simulink model "MIPI"  (R2025a)
settings: Solver=ode1  StartTime=0.0  StopTime=Ttotal  FixedStep=Tsample  MaxStep=1e-3  RelTol=1e-3
values from neighbouring files (symbols this model uses):
  A_0 = 1.5762    [Para_PV.m]
  alpha_T = 0.048/100    (= 0.00048)    [Para_PV.m]
  beta_T = -0.32/100    (= -0.0032)    [Para_PV.m]
  Ee = 1    [Para_PV.m]
  gamma = -0.0528    [Para_PV.m]
  Iscs = Iscs    (= 8.7)    [Para_PV.m]
  Np = 1    [Para_PV.m]
  Ns = 60    [Para_PV.m]
  qk0 = 11594    [Para_PV.m]
  Tc = 25    [Para_PV.m]
  Ttotal = 5e-1    (= 0.5)    [Batch_Run_MIPI.m]
  Vocs = Vocs/Ns    (= 0.623333333333)    [Para_PV.m]
settings Model: Creator=mwxiao  LastModifiedBy=yvenk
settings SolverCC: AlgebraicLoopSolver=TrustRegion
settings DataIOCC: LimitDataPoints=on  SaveFormat=Array  SignalLoggingSaveFormat=ModelDataLogs  ReturnWorkspaceOutputs=off  SignalLoggingName=sigsOut
settings OptimizationCC: ExpressionDepthLimit=2147483647.0  LifeSpan=inf
settings DebuggingCC: SaveWithParameterizedLinksMsg=none  UnderspecifiedInitializationDetection=Classic  MergeDetectMultiDrivingBlocksExec=none  SignalResolutionControl=TryResolveAllWithWarning  MultiTaskDSMMsg=warning  MultiTaskCondExecSysMsg=none  FcnCallInpInsideContextMsg=warning  UnconnectedInputMsg=warning  UnconnectedOutputMsg=warning  UnconnectedLineMsg=warning  StateNameClashWarn=warning  SFUnexpectedBacktrackingDiag=warning  SFNoUnconditionalDefaultTransitionDiag=warning  SFExecutionAtInitializationDiag=none  ArithmeticOperatorsInVariantConditions=warning
settings HardwareCC: ProdBitPerPointer=32.0  ProdBitPerSizeT=32.0  ProdBitPerPtrDiffT=32.0  ProdLargestAtomicFloat=None  ProdIntDivRoundTo=Undefined  ProdEndianess=Unspecified  ProdWordSize=32.0  ProdHWDeviceType=32-bit Generic  TargetBitPerPointer=64.0  TargetBitPerSizeT=64.0  TargetBitPerPtrDiffT=64.0  TargetLongLongMode=on  TargetIntDivRoundTo=Zero  TargetEndianess=LittleEndian  TargetWordSize=64.0  TargetHWDeviceType=MATLAB Host  ProdEqTarget=off
settings ModelReferenceCC: EnableRefExpFcnMdlSchedulingChecks=on  PropagateSignalLabelsOutOfModel=off
settings SFSimCC: SimUseLocalCustomCode=off  CustomCodeUndefinedFunction=UseInterfaceOnly
settings RTWCC: RTWUseLocalCustomCode=off  GPUComputeCapability=3.5  DLArmComputeVersion=19.05
settings CodeAppCC: StateflowObjectComments=on
settings GRTTargetCC: TargetLangStandard=C89/C90 (ANSI)  CombineOutputUpdateFcns=off  GRTInterface=on
settings ConfigComp: CovMetricSettings=dw  CovSaveCumulativeToWorkspaceVar=on  CovSaveSingleToWorkspaceVar=on  CovExternalEMLEnable=off

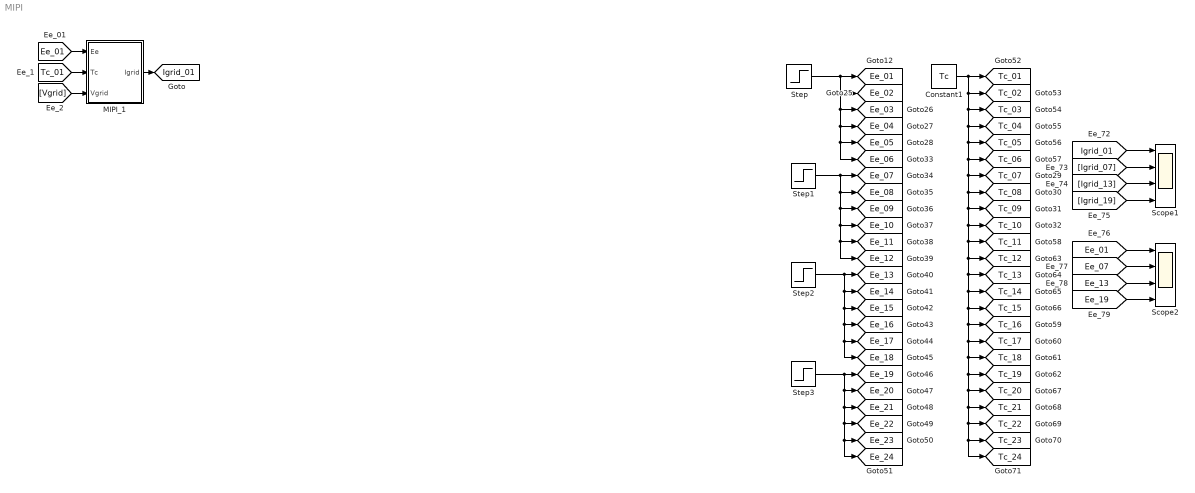
== system MIPI ==
  Constant1 : Constant  Value=Tc
  MIPI_1 : Subsystem
  Scope1 : Scope  NumInputPorts=4
      settings: ActiveDisplayYMinimum=-1.5  ActiveDisplayYMaximum=1.5  DataLoggingVariableName=simout
  Scope2 : Scope  NumInputPorts=4
      settings: ActiveDisplayYMinimum=-1.5  ActiveDisplayYMaximum=1.5  DataLoggingVariableName=simout1
  Step : Step  Time=Ttotal/2+0.005  Before=Ee*0.9  After=Ee*0.7  SampleTime=0
  Step1 : Step  Time=Ttotal/2+0.005  Before=Ee*0.8  After=Ee*0.6  SampleTime=0
  Step2 : Step  Time=Ttotal/2+0.005  Before=Ee*0.7  After=Ee*0.5  SampleTime=0
  Step3 : Step  Time=Ttotal/2+0.005  Before=Ee*0.6  After=Ee*0.8  SampleTime=0
  tag scope: Ee_01=global, Ee_02=global, Ee_03=global, Ee_04=global, Ee_05=global, Ee_06=global, Ee_07=global, Ee_08=global, Ee_09=global, Ee_10=global, Ee_11=global, Ee_12=global, Ee_13=global, Ee_14=global, Ee_15=global, Ee_16=global, Ee_17=global, Ee_18=global, Ee_19=global, Ee_20=global, Ee_21=global, Ee_22=global, Ee_23=global, Ee_24=global, Igrid_01=global, Tc_01=global, Tc_02=global, Tc_03=global, Tc_04=global, Tc_05=global, Tc_06=global, Tc_07=global, Tc_08=global, Tc_09=global, Tc_10=global, Tc_11=global, Tc_12=global, Tc_13=global, Tc_14=global, Tc_15=global, Tc_16=global, Tc_17=global, Tc_18=global, Tc_19=global, Tc_20=global, Tc_21=global, Tc_22=global, Tc_23=global, Tc_24=global
  wires:
  [Ee_13] -> Scope2/3
  [Ee_19] -> Scope2/4
  Step1/1 -> [Ee_11], [Ee_12], [Ee_10], [Ee_09], [Ee_08], [Ee_07]
  [Igrid_13] -> Scope1/3
  [Ee_01] -> Scope2/1
  [Igrid_01] -> Scope1/1
  [Igrid_19] -> Scope1/4
  [Ee_07] -> Scope2/2
  [Igrid_07] -> Scope1/2
  Step/1 -> [Ee_01], [Ee_03], [Ee_04], [Ee_05], [Ee_06], [Ee_02]
  Constant1/1 -> [Tc_08], [Tc_17], [Tc_18], [Tc_21], [Tc_22], [Tc_23], [Tc_24], [Tc_20], [Tc_19], [Tc_16], [Tc_15], [Tc_14], [Tc_13], [Tc_12], [Tc_11], [Tc_10], [Tc_09], [Tc_07], [Tc_06], [Tc_05], [Tc_04], [Tc_03], [Tc_02], [Tc_01]
  Step3/1 -> [Ee_23], [Ee_24], [Ee_22], [Ee_21], [Ee_20], [Ee_19]
  Step2/1 -> [Ee_17], [Ee_18], [Ee_16], [Ee_15], [Ee_14], [Ee_13]
  [Vgrid] -> MIPI_1/3(Vgrid)
  [Tc_01] -> MIPI_1/2(Tc)
  [Ee_01] -> MIPI_1/1(Ee)
  MIPI_1/1(Igrid) -> [Igrid_01]

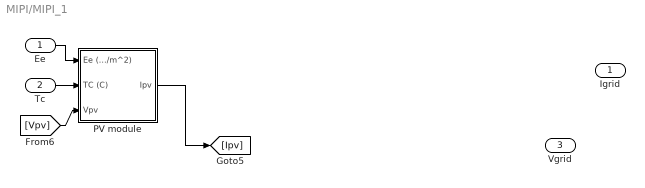
== system MIPI/MIPI_1 ==
  Ee : Inport
  Tc : Inport  Port=2
  Vgrid : Inport  Port=3
  PV module : Subsystem
  Igrid : Outport
  wires:
  [Vpv] -> PV module/3(Vpv)
  PV module/1(Ipv) -> [Ipv]
  Ee/1 -> PV module/1(Ee (1kW/m^2))
  Tc/1 -> PV module/2(TC (C))

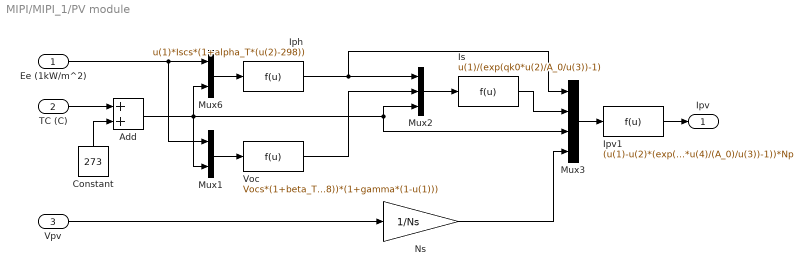
== system MIPI/MIPI_1/PV module ==
  Ee (1kW/m^2) : Inport
  TC (C) : Inport  Port=2
  Vpv : Inport  Port=3
  Add : Sum
  Constant : Constant  Value=273
  Iph : Fcn  Expr=u(1)*Iscs*(1+alpha_T*(u(2)-298))
  Ipv1 : Fcn  Expr=(u(1)-u(2)*(exp(qk0*u(4)/(A_0)/u(3))-1))*Np
  Is : Fcn  Expr=u(1)/(exp(qk0*u(2)/A_0/u(3))-1)
  Mux1 : Mux  Inputs=2
  Mux2 : Mux  Inputs=3
  Mux3 : Mux
  Mux6 : Mux  Inputs=2
  Ns : Gain  Gain=1/Ns
  Voc : Fcn  Expr=Vocs*(1+beta_T*(u(2)-298))*(1+gamma*(1-u(1)))
  Ipv : Outport
  wires:
  Mux6/1 -> Iph/1
  Ee (1kW/m^2)/1 -> Mux6/1, Mux1/1
  Mux1/1 -> Voc/1
  Mux2/1 -> Is/1
  Iph/1 -> Mux2/1, Mux3/1
  Voc/1 -> Mux2/2
  Mux3/1 -> Ipv1/1
  Is/1 -> Mux3/2
  Vpv/1 -> Ns/1
  Ipv1/1 -> Ipv/1
  TC (C)/1 -> Add/1
  Add/1 -> Mux6/2, Mux1/2, Mux2/3, Mux3/3
  Constant/1 -> Add/2
  Ns/1 -> Mux3/4
